simulink model "otch_5_3l"  (R2017b)
settings: Solver=VariableStepAuto  StartTime=0.0  StopTime=0.6  RelTol=1e-3
values from neighbouring files (symbols this model uses):
  g1 = G(1), g2=G(2)    [fin_helper.m]    (also in kriter.m = G(1))
  g2 = G(2)    [kriter.m]
settings Model: Creator=anton  LastModifiedBy=HONOR

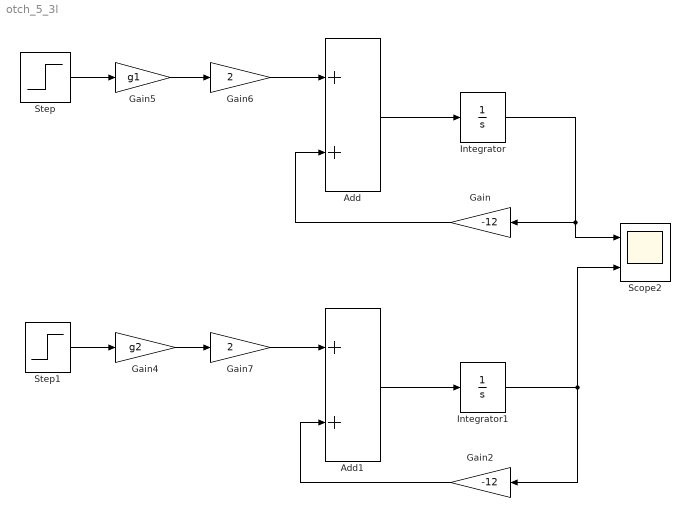
== system otch_5_3l ==
  Add : Sum
  Add1 : Sum
  Gain : Gain  Gain=-12
  Gain2 : Gain  Gain=-12
  Gain4 : Gain  Gain=g2
  Gain5 : Gain  Gain=g1
  Gain6 : Gain  Gain=2
  Gain7 : Gain  Gain=2
  Integrator : Integrator
  Integrator1 : Integrator
  Scope2 : Scope  NumInputPorts=2
  Step : Step  Time=0  After=1.9  SampleTime=0
  Step1 : Step  Time=0  After=1.9  SampleTime=0
  wires:
  Add/1 -> Integrator/1
  Integrator/1 -> Scope2/1, Gain/1
  Integrator1/1 -> Scope2/2, Gain2/1
  Add1/1 -> Integrator1/1
  Step1/1 -> Gain4/1
  Step/1 -> Gain5/1
  Gain5/1 -> Gain6/1
  Gain6/1 -> Add/1
  Gain7/1 -> Add1/1
  Gain/1 -> Add/2
  Gain4/1 -> Gain7/1
  Gain2/1 -> Add1/2
